simulink model "Model"  (R2018a)
settings: Solver=ode45  StartTime=0.0  StopTime=5  MaxStep=0.001  RelTol=1e-3
settings Model: Creator=LAKE  LastModifiedBy=LAKE

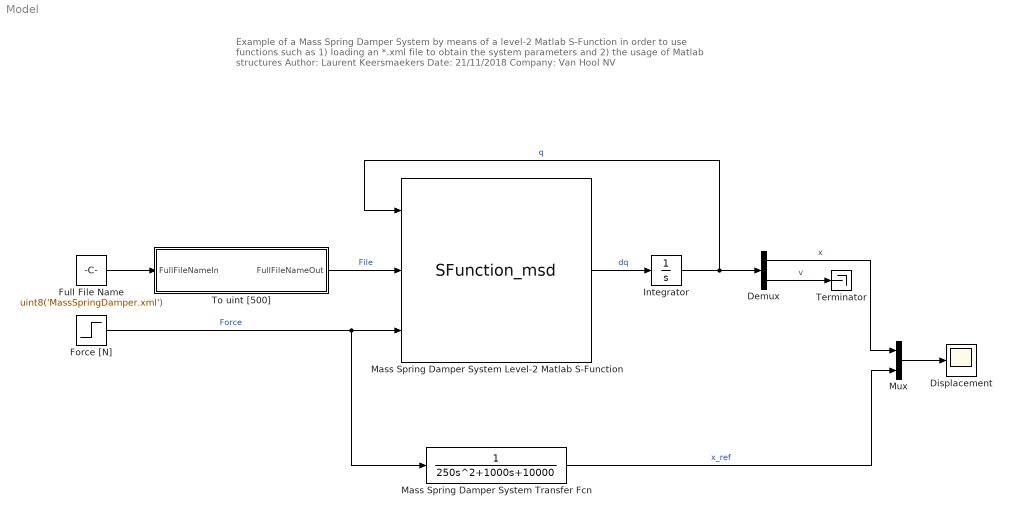
== system Model ==
  note: Example of a Mass Spring Damper System by means of a level-2 Matlab S-Function in order to use functions such as
      |   1) loading an *.xml file to obtain the system parameters and
      |   2) the usage of Matlab structures
      |
      | Author: 		Laurent Keersmaekers
      | Date:		21/11/2018
      | Company:	Van Hool NV
  Demux : Demux  Outputs=2
  Displacement : Scope
  Force [N] : Step  After=10000  SampleTime=0
  Full File Name : Constant  Value=uint8('MassSpringDamper.xml')  OutDataTypeStr=Inherit: Inherit via back propagation
  Integrator : Integrator  InitialCondition=[0 0]
  Mass Spring Damper System Level-2 Matlab S-Function : M-S-Function  FunctionName=SFunction_msd
      mask Display:
      | port_label('input', 1, 'q');
      | port_label('input', 2, 'Full File Name');
      | port_label('output', 1, 'dq');
      | fprintf('MSD')
  Mass Spring Damper System Transfer Fcn : TransferFcn  Denominator=[250 1000 10000]
  Mux : Mux  Inputs=2
  Terminator : Terminator
  To uint [500] : MATLAB Function  TreatAsAtomicUnit=on
  wires:
  Mass Spring Damper System Level-2 Matlab S-Function/1 -> Integrator/1  "dq"
  Integrator/1 -> Demux/1, Mass Spring Damper System Level-2 Matlab S-Function/1  "q"
  Full File Name/1 -> To uint [500]/1(FullFileNameIn)
  To uint [500]/1(FullFileNameOut) -> Mass Spring Damper System Level-2 Matlab S-Function/2  "File"
  Force [N]/1 -> Mass Spring Damper System Transfer Fcn/1, Mass Spring Damper System Level-2 Matlab S-Function/3  "Force"
  Demux/1 -> Mux/1  "x"
  Mass Spring Damper System Transfer Fcn/1 -> Mux/2  "x_ref"
  Mux/1 -> Displacement/1
  Demux/2 -> Terminator/1  "v"

== matlab function Model/To uint [500] ==
  data: FullFileNameIn input; FullFileNameOut output
function FullFileNameOut = fcn(FullFileNameIn)

% This function converts a variable length uint8 variable into a uint8
% variable containing 500 elements. This is required (?) as an input for
% the Level-2 Matlab S-function

% Author:  Laurent Keersmaekers
% Date:    21/11/2018
% Company: Van Hool NV

uint8_500               = uint8(char(32*ones(1,500)));
uint8_500(...
  1:length(...
    FullFileNameIn))    = FullFileNameIn;

FullFileNameOut         = uint8_500;
